simulink model "ClosedLoopTest"  (R2023b)
settings: Solver=FixedStepAuto  StartTime=0.0  StopTime=60  FixedStep=T  MaxStep=0.015  RelTol=1e-3
StopFcn:
  | stopHeli_allTasks
  | daqreset
model workspace: external: MAT-File (data not in the file)
values from neighbouring files (symbols this model uses):
  b = fir1(50, 0.004)    [heli_real.m]
  Cr = [1,0,0,0,0,0 ... (first row only)    [heli_real.m]
  DAC_lim_l = 0    [heli_real.m]
  DAC_lim_u = 10    [heli_real.m]
  e_lim_l = min(ElevAxisData.Var1)*pi/180    [heli_real.m]
  ElevAxisData = readtable('ElevAxisData.txt')    [heli_real.m]
  K = Kaug(:,1:6)    [heli_real.m]
  ki = -Kaug(:,7:8)    [heli_real.m]
  PitchAxisData = readtable('PitchAxisData.txt')    [heli_real.m]
  T = 0.03    [heli_real.m]
  U_e = 5.5    [heli_real.m]
undefined symbols (not defined in the file or in its folder): DiscIntNeverNeededParam, kdfilt
libraries: sldrtlib x1
settings Model: Creator=msciola  LastModifiedBy=GCRAFT
settings SolverCC: AlgebraicLoopSolver=TrustRegion
settings DebuggingCC: UnconnectedInputMsg=warning  UnconnectedOutputMsg=warning  UnconnectedLineMsg=warning
settings ModelReferenceCC: EnableRefExpFcnMdlSchedulingChecks=on
settings SFSimCC: CustomCodeUndefinedFunction=UseInterfaceOnly

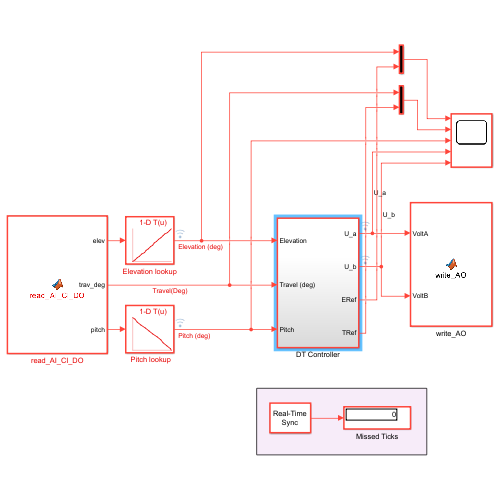
[thumbnail: Simulink's stored preview of the top-level diagram]
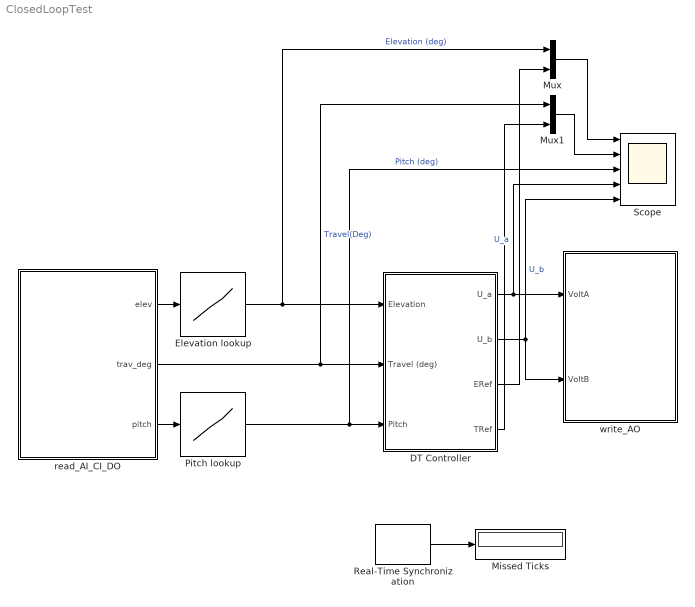
== system ClosedLoopTest ==
  " Pitch lookup" : Lookup_n-D  NumberOfTableDimensions=1  LookupTableObject=PitchAxisData  BreakpointsForDimension1=PitchAxisData.Var2  Table=PitchAxisData.Var1  InternalRulePriority=Speed  RndMeth=Simplest
  DT Controller : Subsystem
  Elevation lookup : Lookup_n-D  NumberOfTableDimensions=1  LookupTableObject=PitchAxisData  BreakpointsForDimension1=ElevAxisData.Var2  Table=ElevAxisData.Var1  InternalRulePriority=Speed  RndMeth=Simplest
  Missed Ticks : Display
  Mux : Mux  Inputs=2
  Mux1 : Mux  Inputs=2
  Real-Time Synchronization : sldrtlib/Real-Time Synchronization  SampleTime=T  MaxMissedTicks=inf  ShowMissedTicks=on  YieldWhenWaiting=off
  Scope : Scope  NumInputPorts=5
  read_AI_CI_DO : MATLAB Function  TreatAsAtomicUnit=on
  write_AO : MATLAB Function  TreatAsAtomicUnit=on
  wires:
  Real-Time Synchronization/1 -> Missed Ticks/1
  read_AI_CI_DO/2(trav_deg) -> Mux1/1, DT Controller/2(Travel (deg))  "Travel(Deg)"
  DT Controller/1(U_a) -> write_AO/1(VoltA), Scope/4  "U_a"
  read_AI_CI_DO/1(elev) -> Elevation lookup/1
  Elevation lookup/1 -> Mux/1, DT Controller/1(Elevation)  "Elevation (deg)"
  read_AI_CI_DO/3(pitch) -> " Pitch lookup"/1
  " Pitch lookup"/1 -> Scope/3, DT Controller/3(Pitch)  "Pitch (deg)"
  DT Controller/2(U_b) -> write_AO/2(VoltB), Scope/5  "U_b"
  DT Controller/3(ERef) -> Mux/2
  Mux/1 -> Scope/1
  DT Controller/4(TRef) -> Mux1/2
  Mux1/1 -> Scope/2

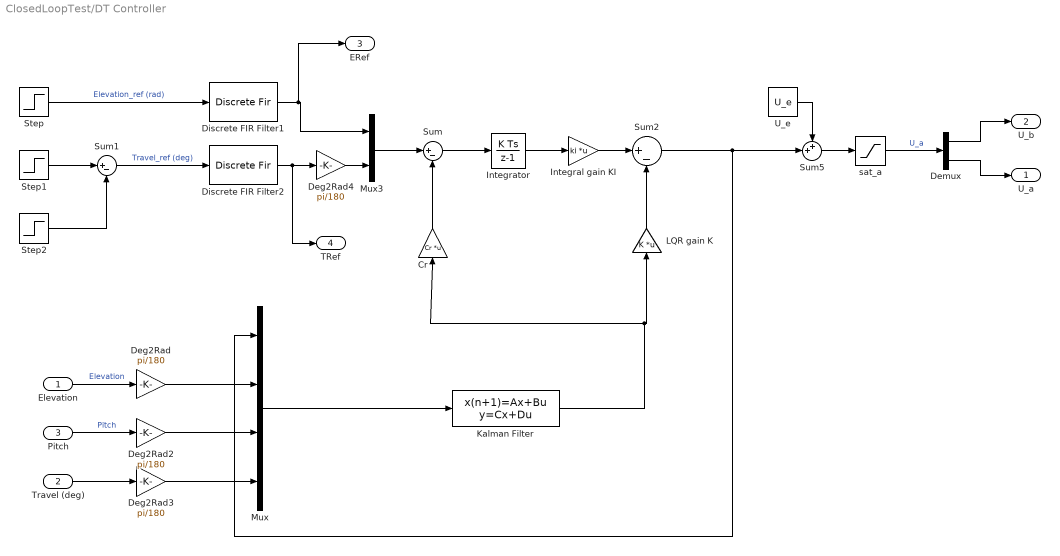
== system ClosedLoopTest/DT Controller ==
  Elevation : Inport
  Travel (deg) : Inport  Port=2
  Pitch : Inport  Port=3
  Cr : Gain  Gain=Cr  Multiplication=Matrix(K*u)
  Deg2Rad{,2..4} (4 alike) : Gain  Gain=pi/180
  Demux : Demux  Outputs=2
  Discrete FIR Filter1 : DiscreteFir  Coefficients=b  InputProcessing=Columns as channels (frame based)
  Discrete FIR Filter2 : DiscreteFir  Coefficients=b  InputProcessing=Columns as channels (frame based)
  Integral gain KI : Gain  Gain=ki  Multiplication=Matrix(K*u)
  Integrator : DiscreteIntegrator  SampleTime=T  ICPrevOutput=DiscIntNeverNeededParam  ICPrevScaledInput=DiscIntNeverNeededParam
  Kalman Filter : DiscreteStateSpace  A=kdfilt.a  B=kdfilt.b  C=kdfilt.c(size(C,1)+1:end,:)  D=kdfilt.d(size(C,1)+1:end,:)  InitialCondition=[e_lim_l; 0; 0; 0; 0; 0]  SampleTime=T
  LQR gain K : Gain  Gain=K  Multiplication=Matrix(K*u)
  Mux : Mux
  Mux3 : Mux  Inputs=2
  Step : Step  Time=0  Before=e_lim_l  After=0  SampleTime=T
  Step1 : Step  Time=20  After=180  SampleTime=T
  Step2 : Step  Time=40  After=180  SampleTime=T
  Sum : Sum  Inputs=|+-
  Sum1 : Sum  Inputs=|+-
  Sum2 : Sum  Inputs=|+-
  Sum5 : Sum  Inputs=++|
  U_e : Constant  Value=U_e  SampleTime=T
  sat_a : Saturate  UpperLimit=DAC_lim_u  LowerLimit=DAC_lim_l
  U_a : Outport
  U_b : Outport  Port=2
  ERef : Outport  Port=3
  TRef : Outport  Port=4
  wires:
  Travel (deg)/1 -> Deg2Rad3/1
  Sum/1 -> Integrator/1
  Mux3/1 -> Sum/1
  Sum2/1 -> Sum5/2, Mux/1
  LQR gain K/1 -> Sum2/2
  Cr/1 -> Sum/2
  Kalman Filter/1 -> Cr/1, LQR gain K/1
  Pitch/1 -> Deg2Rad2/1  "Pitch"
  Integral gain KI/1 -> Sum2/1
  Elevation/1 -> Deg2Rad/1  "Elevation"
  Mux/1 -> Kalman Filter/1
  U_e/1 -> Sum5/1
  Integrator/1 -> Integral gain KI/1
  Deg2Rad4/1 -> Mux3/2
  Deg2Rad/1 -> Mux/2
  Deg2Rad2/1 -> Mux/3
  Deg2Rad3/1 -> Mux/4
  Sum5/1 -> sat_a/1
  Discrete FIR Filter2/1 -> TRef/1, Deg2Rad4/1
  Step1/1 -> Sum1/1
  Step2/1 -> Sum1/2
  Sum1/1 -> Discrete FIR Filter2/1  "Travel_ref (deg)"
  Step/1 -> Discrete FIR Filter1/1  "Elevation_ref (rad)"
  Discrete FIR Filter1/1 -> ERef/1, Mux3/1
  sat_a/1 -> Demux/1  "U_a"
  Demux/1 -> U_b/1
  Demux/2 -> U_a/1

== matlab function ClosedLoopTest/read_AI_CI_DO ==
  data: elev output; trav_deg output; pitch output
function [elev,trav_deg,pitch] = read_AI_CI_DO()
% The functions from the NI library to read and write inputs and outpus 
% cannot be compiled and we need to use the coder.extrinsic.
% Functions in common to all 
coder.extrinsic('NI_DAQmxCreateTask','NI_DAQmxStartTask','assignin');
%Functions to read AI
coder.extrinsic('daq.ni.NIDAQmx.DAQmx_Val_Diff','NI_DAQmxCreateAIVoltageChan',...
    'NI_DAQmxReadAnalogF64');
%Functions to read CI
coder.extrinsic('NI_DAQmxCreateCILinEncoderChan','NI_DAQmxReadCounterScalarF64',... 
    'daq.ni.NIDAQmx.DAQmx_Val_X1','daq.ni.NIDAQmx.DAQmx_Val_Ticks');
%Functions to write DO
coder.extrinsic('NI_DAQmxWriteDigitalLines','NI_DAQmxCreateDOChan');

%% Configuration
% Specify channels
channelNameAI = {'myDAQ1/ai0','myDAQ1/ai1'};
channelNameCI = 'myDAQ1/ctr0';
channelNamesDO = {'myDAQ1/Port0/Line5', 'myDAQ1/Port0/Line6','myDAQ1/Port0/Line7'};

% Initialize variables for MATLAB Function block to work
elev = 0;
pitch = 0;
numChannels = 1;
trav = zeros(1, numChannels);
y = zeros(1, numChannels);
% make the taskhandle for each channel persistent
persistent taskHandleAI taskHandleCI taskHandleDO
% Create and start tasks for each channel
if isempty(taskHandleAI)
    taskHandleAI = NI_DAQmxCreateTask;
    NI_DAQmxCreateAIVoltageChan(taskHandleAI, channelNameAI{1}, daq.ni.NIDAQmx.DAQmx_Val_Diff, -10, 10)
    NI_DAQmxCreateAIVoltageChan(taskHandleAI, channelNameAI{2}, daq.ni.NIDAQmx.DAQmx_Val_Diff, -10, 10)
    NI_DAQmxStartTask(taskHandleAI);
    assignin('base','taskHandleAI',taskHandleAI);
end
if isempty(taskHandleCI)
    taskHandleCI = NI_DAQmxCreateTask;
    NI_DAQmxCreateCILinEncoderChan( taskHandleCI, channelNameCI, daq.ni.NIDAQmx.DAQmx_Val_X1, daq.ni.NIDAQmx.DAQmx_Val_Ticks, 1); % Check X4 (Labview) or X1 with Bryn
    NI_DAQmxStartTask(taskHandleCI)
    assignin('base','taskHandleCI',taskHandleCI);
end
if isempty (taskHandleDO)
    taskHandleDO = NI_DAQmxCreateTask;
    for ii = 1:numel(channelNamesDO)
        NI_DAQmxCreateDOChan(taskHandleDO, channelNamesDO{ii});
    end
    %numChannelsDO = NI_DAQmxGetWriteNumChans(taskHandleDO);
    NI_DAQmxStartTask(taskHandleDO)
    assignin('base','taskHandleDO',taskHandleDO);
end
%% Read and write channels
% Write the digital outputs
outputData = [0 1 0];
NI_DAQmxWriteDigitalLines(taskHandleDO, outputData);
% Read analog inputs (elevation and pitch angles)
data = NI_DAQmxReadAnalogF64(taskHandleAI,1,2);
elev = data(1);
pitch = data(2);

% Read the counter encoder input (tavel angle)
y = NI_DAQmxReadCounterScalarF64(taskHandleCI);
% To avoid insignificant numbers in the reading
if y> 2^31
    y = y- 2^32;
end
% Transform the encoder reading into angle degrees between 0 and 360
 trav_deg = y*360/500;

== matlab function ClosedLoopTest/write_AO ==
  data: VoltA input; VoltB input
function write_AO(VoltA,VoltB)
% The functions from the NI library to write outpus cannot be compiled 
% and we need to use the coder.extrinsic.
% Functions in common to all  
coder.extrinsic('NI_DAQmxCreateTask','NI_DAQmxStartTask', 'assignin');
% Functions to write AO
coder.extrinsic('NI_DAQmxCreateAOVoltageChan','NI_DAQmxWriteAnalogF64',...
    'daq.ni.NIDAQmx.DAQmx_Val_Volts');
%% Configuration
% Specify channel
channelNameAO = {'myDAQ1/ao0','myDAQ1/ao1'};
% make the taskhandle persistent
persistent  taskHandleAO 
% Create and start tasks for each channel
if isempty(taskHandleAO)
    taskHandleAO = NI_DAQmxCreateTask;
    NI_DAQmxCreateAOVoltageChan(taskHandleAO, channelNameAO{1})
    NI_DAQmxCreateAOVoltageChan(taskHandleAO, channelNameAO{2})
    NI_DAQmxStartTask(taskHandleAO);
    assignin('base','taskHandleAO',taskHandleAO);
end
%% Write Digital output
NI_DAQmxWriteAnalogF64(taskHandleAO,[VoltA,VoltB]);
end
